simulink model "Simulink"  (R2021a)
settings: Solver=FixedStepAuto  StartTime=0.0  StopTime=0.001  FixedStep=1e-8  RelTol=1e-3
undefined symbols (not defined in the file): fdesignblkfcn, gcbh
libraries: dspsigops x2, dspfdesign x2, commchan3 x1
settings Model: Creator=Mario  LastModifiedBy=Mario

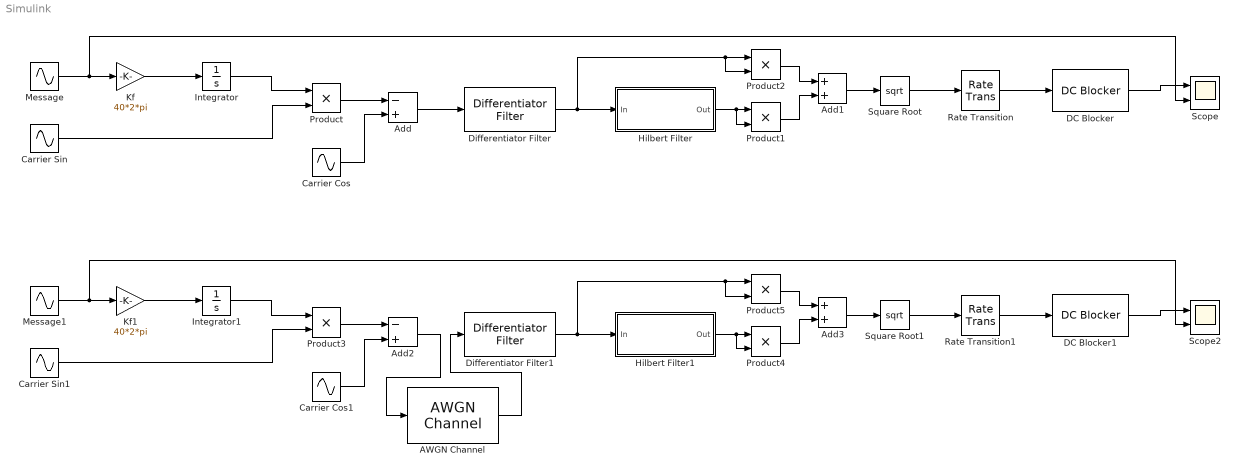
== system Simulink ==
  AWGN Channel : commchan3/AWGN Channel  InputProcessing=Columns as channels (frame based)  seed=67  noiseMode="Signal to noise ratio  (Eb/No)"  EbNodB=100  EsNodB=10  SNRdB=10  bitsPerSym=1  Ps=1  Tsym=1  variance=1
  Add : Sum  Inputs=-+
  Add1 : Sum
  Add2 : Sum  Inputs=-+
  Add3 : Sum
  Carrier Cos : Sin  Frequency=2*pi*90000000  Phase=pi/2  SampleTime=0
  Carrier Cos1 : Sin  Frequency=2*pi*90000000  Phase=pi/2  SampleTime=0
  Carrier Sin : Sin  Frequency=2*pi*90000000  Phase=pi/2  SampleTime=0
  Carrier Sin1 : Sin  Frequency=2*pi*90000000  Phase=pi/2  SampleTime=0
  DC Blocker : dspsigops/DC Blocker  Algorithm=IIR  NormalizedBandwidth=0.001  Length=8  Order=6  SimulateUsing=Code generation
      settings: SourceProductBaseCode=DS
  DC Blocker1 : dspsigops/DC Blocker  Algorithm=IIR  NormalizedBandwidth=0.001  Length=8  Order=6  SimulateUsing=Code generation
      settings: SourceProductBaseCode=DS
  Differentiator Filter : dspfdesign/Differentiator Filter  DesignForMinimumOrder=on  FilterOrder=31  PassbandRipple=0.1  ScaleCoefficients=off  SimulateUsing=Interpreted execution  roundingMode=Floor  coeffsDataTypeStr=fixdt(1,16)
      settings: SourceProductBaseCode=DS
  Differentiator Filter1 : dspfdesign/Differentiator Filter  DesignForMinimumOrder=on  FilterOrder=31  PassbandRipple=0.1  ScaleCoefficients=off  SimulateUsing=Interpreted execution  roundingMode=Floor  coeffsDataTypeStr=fixdt(1,16)
      settings: SourceProductBaseCode=DS
  Hilbert Filter : Subsystem  DialogController=fdesignblkfcn  InitFcn=fdesignblkfcn(gcbh, {'InitFcn'});  mask(Hilbert Filter){}
      mask help: Design a Hilbert filter
      settings: CopyFcn=fdesignblkfcn(gcbh, {'CopyFcn'});
      mask Help: helpview(mapfilelocation('dsp'), 'dsphilbertfilter');
      mask Display: disp('Hilbert')
  Hilbert Filter1 : Subsystem  DialogController=fdesignblkfcn  InitFcn=fdesignblkfcn(gcbh, {'InitFcn'});  mask(Hilbert Filter){}
      mask help: Design a Hilbert filter
      settings: CopyFcn=fdesignblkfcn(gcbh, {'CopyFcn'});
      mask Help: helpview(mapfilelocation('dsp'), 'dsphilbertfilter');
      mask Display: disp('Hilbert')
  Integrator : Integrator
  Integrator1 : Integrator
  Kf : Gain  Gain=40*2*pi
  Kf1 : Gain  Gain=40*2*pi
  Message : Sin  Frequency=2*pi*1000  Phase=pi/2  SampleTime=0
  Message1 : Sin  Frequency=2*pi*1000  Phase=pi/2  SampleTime=0
  Product{,1..5} (6 alike) : Product
  Rate Transition : RateTransition  OutPortSampleTimeMultiple=0.0001
  Rate Transition1 : RateTransition  OutPortSampleTimeMultiple=0.0001
  Scope : Scope  NumInputPorts=2
  Scope2 : Scope  NumInputPorts=2
  Square Root : Sqrt  SaturateOnIntegerOverflow=on
  Square Root1 : Sqrt  SaturateOnIntegerOverflow=on
  wires:
  Kf/1 -> Integrator/1
  Integrator/1 -> Product/1
  Carrier Sin/1 -> Product/2
  Product/1 -> Add/1
  Carrier Cos/1 -> Add/2
  Add/1 -> Differentiator Filter/1
  Message/1 -> Scope/2, Kf/1
  Product2/1 -> Add1/1
  Product1/1 -> Add1/2
  Add1/1 -> Square Root/1
  Differentiator Filter/1 -> Product2/2, Product2/1, Hilbert Filter/1(In)
  Hilbert Filter/1(Out) -> Product1/2, Product1/1
  Square Root/1 -> Rate Transition/1
  Rate Transition/1 -> DC Blocker/1
  DC Blocker/1 -> Scope/1
  Add3/1 -> Square Root1/1
  Hilbert Filter1/1(Out) -> Product4/2, Product4/1
  Square Root1/1 -> Rate Transition1/1
  Product4/1 -> Add3/2
  DC Blocker1/1 -> Scope2/1
  Rate Transition1/1 -> DC Blocker1/1
  Carrier Cos1/1 -> Add2/2
  Product5/1 -> Add3/1
  Product3/1 -> Add2/1
  Differentiator Filter1/1 -> Product5/2, Product5/1, Hilbert Filter1/1(In)
  Kf1/1 -> Integrator1/1
  Integrator1/1 -> Product3/1
  Message1/1 -> Scope2/2, Kf1/1
  Carrier Sin1/1 -> Product3/2
  Add2/1 -> AWGN Channel/1
  AWGN Channel/1 -> Differentiator Filter1/1

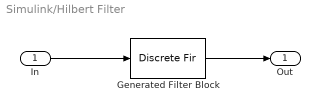
== system Simulink/Hilbert Filter ==
  In : Inport
  Generated Filter Block : DiscreteFir  Tag=BlockMethodSubSystem  Coefficients=[-0.026449858259791379 -0.00578355491829027 -0.016572261903348456 -0.0095390561131982743 -0.022461390535071568 -0.014999256435125952 -0.030323967074738556 -0.023012528163449009 -0.041429315821655127 -0.035762828939278346 -0.05911752381753177 -0.059034685410808696 -0.094459906652176406 -0.11739830204172252 -0.21797718993610349 -0.62869353747279177 0.62869353747279177 0.21797718993610349 0.11739830204172252 0.094459906652176406 0.059034685410808696 0.05911752381753177 0.035762828939278346 0.041429315821655127 0.023012528163449009 0.030323967074738556 0.014999256435125952 0.022461390535071568 0.0095390561131982743 0.016572261903348456 0.00578355491829027 0.026449858259791379]  InputProcessing=Columns as channels (frame based)
  Out : Outport  VectorParamsAs1DForOutWhenUnconnected=off
  wires:
  Generated Filter Block/1 -> Out/1
  In/1 -> Generated Filter Block/1

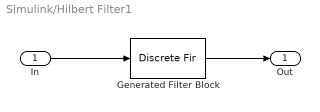
== system Simulink/Hilbert Filter1 ==
  In : Inport
  Generated Filter Block : DiscreteFir  Tag=BlockMethodSubSystem  Coefficients=[-0.026449858259791379 -0.00578355491829027 -0.016572261903348456 -0.0095390561131982743 -0.022461390535071568 -0.014999256435125952 -0.030323967074738556 -0.023012528163449009 -0.041429315821655127 -0.035762828939278346 -0.05911752381753177 -0.059034685410808696 -0.094459906652176406 -0.11739830204172252 -0.21797718993610349 -0.62869353747279177 0.62869353747279177 0.21797718993610349 0.11739830204172252 0.094459906652176406 0.059034685410808696 0.05911752381753177 0.035762828939278346 0.041429315821655127 0.023012528163449009 0.030323967074738556 0.014999256435125952 0.022461390535071568 0.0095390561131982743 0.016572261903348456 0.00578355491829027 0.026449858259791379]  InputProcessing=Columns as channels (frame based)
  Out : Outport  VectorParamsAs1DForOutWhenUnconnected=off
  wires:
  Generated Filter Block/1 -> Out/1
  In/1 -> Generated Filter Block/1
